simulink model "ShapesDemo"  (R2022b)
settings: Solver=FixedStepAuto  StartTime=0.0  StopTime=inf  RelTol=1e-3
libraries: ddsblock x2
settings Model: DataDictionary=ShapesDemo.sldd  Creator=tamli  LastModifiedBy=tamli
settings DataIOCC: SaveOutput=off
settings OptimizationCC: DefaultParameterBehavior=Inlined  EnhancedBackFolding=on  PassReuseOutputArgsAs=Individual arguments  ZeroExternalMemoryAtStartup=off  ZeroInternalMemoryAtStartup=off  OptimizeBlockOrder=speed  DifferentSizesBufferReuse=on  OptimizationCustomize=off  EfficientTunableParamExpr=on
settings DebuggingCC: ParameterTunabilityLossMsg=error
settings SFSimCC: SimGenImportedTypeDefs=on  MATLABDynamicMemAlloc=off
settings RTWCC: Description=Embedded Coder  SystemTargetFile=ert.tlc  TemplateMakefile=ert_default_tmf  Toolchain=RTI Connext 6.0 Project  TargetLang=C++
settings CodeAppCC: ForceParamTrailComments=on  IgnoreCustomStorageClasses=off  OperatorAnnotations=on  SimulinkDataObjDesc=on  SFDataObjDesc=on  InsertBlockDesc=on
settings ERTTargetCC: TargetLangStandard=C++11 (ISO)  CodeInterfacePackaging=C++ class  InlinedParameterPlacement=NonHierarchical  RootIOFormat=Structure reference  ERTCustomFileTemplate=example_file_process.tlc  ArrayContainerType=std::array

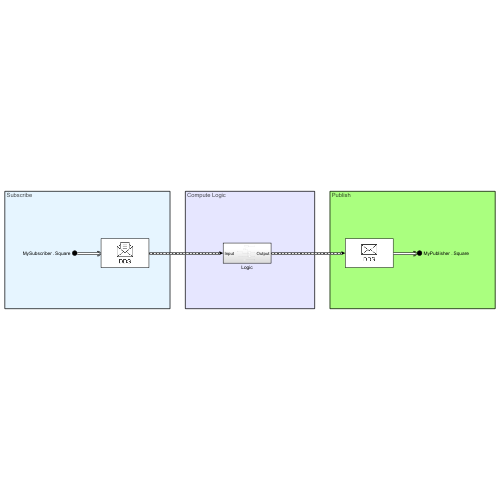
[thumbnail: Simulink's stored preview of the top-level diagram]
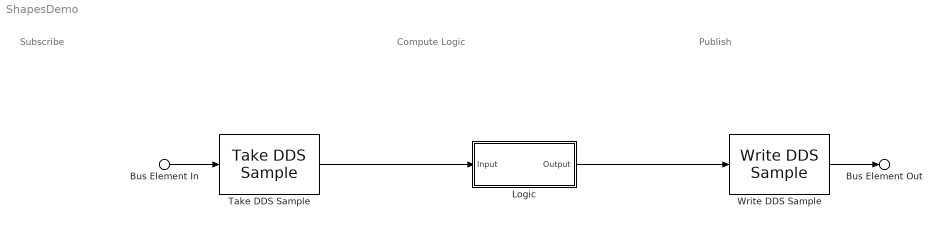
== system ShapesDemo ==
  note: Publish
  note: Compute Logic
  note: Subscribe
  Bus Element In : Inport  PortName=MySubscriber  Element=Square
  Logic : Subsystem
  Take DDS Sample : ddsblock/Take DDS Sample  UseInternalQueue=off  QueueOverwriting=off  QueueLength=16  QueueType=FIFO  PriorityOrder=Ascending  ShowQueueStatus=off  InitialValue=[]  ValueSourceWhenQueueIsEmpty=Use initial value  SampleTime=-1
      settings: LibrarySourceBlock=ddslib/Take DDS Sample
  Write DDS Sample : ddsblock/Write DDS Sample
      settings: LibrarySourceBlock=ddslib/Write DDS Sample
  Bus Element Out : Outport  InputPortMessageModes=m  PortName=MyPublisher  Element=Square
  wires:
  Take DDS Sample/1 -> Logic/1(Input)
  Logic/1(Output) -> Write DDS Sample/1
  Bus Element In/1 -> Take DDS Sample/1
  Write DDS Sample/1 -> Bus Element Out/1

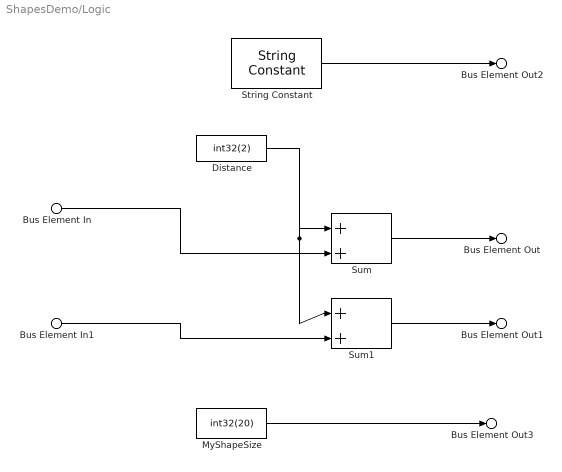
== system ShapesDemo/Logic ==
  Bus Element In : Inport  PortName=Input  Element=x
  Bus Element In1 : Inport  PortName=Input  Element=y
  Distance : Constant  Value=int32(2)
  MyShapeSize : Constant  Value=int32(20)
  String Constant : StringConstant  String="\"Red\""
  Sum : Sum  Inputs=|++
  Sum1 : Sum  Inputs=|++
  Bus Element Out2 : Outport  PortName=Output  Element=color
  Bus Element Out : Outport  PortName=Output  Element=x
  Bus Element Out1 : Outport  PortName=Output  Element=y
  Bus Element Out3 : Outport  PortName=Output  Element=shapesize
  wires:
  Distance/1 -> Sum1/1, Sum/1
  Bus Element In/1 -> Sum/2
  Sum/1 -> Bus Element Out/1
  Bus Element In1/1 -> Sum1/2
  Sum1/1 -> Bus Element Out1/1
  String Constant/1 -> Bus Element Out2/1
  MyShapeSize/1 -> Bus Element Out3/1
